simulink model "close_loop_system"  (Simulink 7.7)
settings: Solver=ode45  StartTime=0.0  StopTime=10.0  RelTol=1e-3
values from neighbouring files (symbols this model uses):
  Jt = 0.002    [BE7_trame.m]
  K = place(sys.a, sys.b(:,1), Pc)    [BE7_trame.m]
  Kci = 1    [BE7_trame.m]
  Kcp = 1    [BE7_trame.m]
  Kcv = 0.0314    [BE7_trame.m]
  Ke = 0.2    [BE7_trame.m]
  Kg = 0.2    [BE7_trame.m]
  Le = 0.002    [BE7_trame.m]
  N = 300    [BE7_trame.m]
  Re = 2    [BE7_trame.m]
libraries: simulink x1
settings Model: Creator=a.pagliai  LastModifiedBy=Anthony
settings DataIOCC: SignalLoggingSaveFormat=Dataset
settings OptimizationCC: ExpressionDepthLimit=128
settings CodeAppCC: CustomSymbolStrType=$N$R$M_T
settings GRTTargetCC: CombineOutputUpdateFcns=on

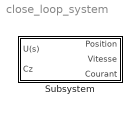
== system close_loop_system ==
  Subsystem : Subsystem

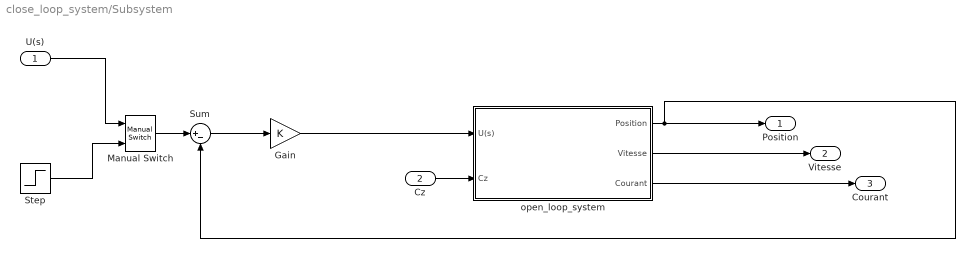
== system close_loop_system/Subsystem ==
  U(s) : Inport
  Cz : Inport  Port=2
  Gain : Gain  Gain=K
  Manual Switch : simulink/Signal Routing/Manual Switch  SystemSampleTime=-1  sw=1  action=0  varsize=off
  Step : Step  SampleTime=0
  Sum : Sum  Inputs=|+-
  "open_loop_system " : Subsystem
  Position : Outport
  Vitesse : Outport  Port=2
  Courant : Outport  Port=3
  wires:
  Cz/1 -> "open_loop_system "/2(Cz)
  "open_loop_system "/1(Position) -> Position/1, Sum/2
  "open_loop_system "/2(Vitesse) -> Vitesse/1
  "open_loop_system "/3(Courant) -> Courant/1
  Sum/1 -> Gain/1
  Gain/1 -> "open_loop_system "/1(U(s))
  Manual Switch/1 -> Sum/1
  U(s)/1 -> Manual Switch/1
  Step/1 -> Manual Switch/2

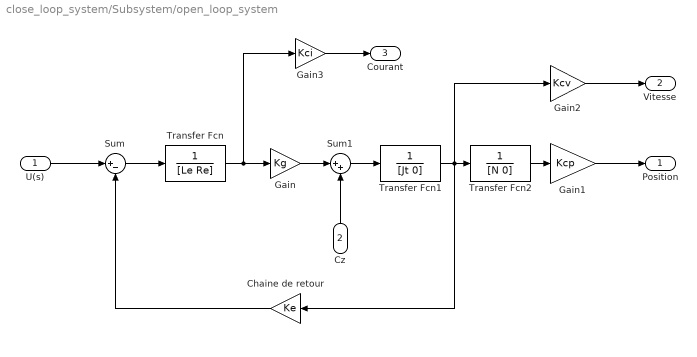
== system close_loop_system/Subsystem/open_loop_system  ==
  U(s) : Inport
  Cz : Inport  Port=2
  Chaine de retour : Gain  Gain=Ke
  Gain : Gain  Gain=Kg
  Gain1 : Gain  Gain=Kcp
  Gain2 : Gain  Gain=Kcv
  Gain3 : Gain  Gain=Kci
  Sum : Sum  Inputs=|+-
  Sum1 : Sum  Inputs=|++
  Transfer Fcn : TransferFcn  Denominator=[Le Re]
  Transfer Fcn1 : TransferFcn  Denominator=[Jt 0]
  Transfer Fcn2 : TransferFcn  Denominator=[N 0]
  Position : Outport
  Vitesse : Outport  Port=2
  Courant : Outport  Port=3
  wires:
  Gain1/1 -> Position/1
  Gain3/1 -> Courant/1
  Gain2/1 -> Vitesse/1
  Cz/1 -> Sum1/2
  U(s)/1 -> Sum/1
  Transfer Fcn2/1 -> Gain1/1
  Chaine de retour/1 -> Sum/2
  Transfer Fcn1/1 -> Chaine de retour/1, Transfer Fcn2/1, Gain2/1
  Transfer Fcn/1 -> Gain/1, Gain3/1
  Sum/1 -> Transfer Fcn/1
  Sum1/1 -> Transfer Fcn1/1
  Gain/1 -> Sum1/1
